simulink model "L20MSDsim"  (R2021b)
settings: Solver=FixedStepAuto  StartTime=0.0  StopTime=10  FixedStep=0.01  RelTol=1e-3
InitFcn:
  | L20ParametersMSD;
values from neighbouring files (symbols this model uses):
  A = [0 1 ; -k/m -b/m]    [L20ParametersMSD.m]    (also in L20ParametersPend.m = [0 1 ; g/l -r/(m*l^2)])
  B = [0 ; 1/m]    [L20ParametersMSD.m]    (also in L20ParametersPend.m = [0 ; 1/(m*l^2)])
  C = [1 0]    [L20ParametersMSD.m]    (also in L20ParametersPend.m)
  eta0 = -L*x0(1)    [L20ParametersMSD.m]    (also in L20ParametersPend.m)
  L = place(A(2,2),A(1,2),-10)    [L20ParametersMSD.m]    (also in L20ParametersPend.m = place(A(2,2),A(1,2),-2))
  x0 = [1; 0.5]    [L20ParametersMSD.m]    (also in L20ParametersPend.m = [theta0 ; thetadot0])
settings Model: Creator=vcichella  LastModifiedBy=vcichella_l
settings SolverCC: AlgebraicLoopSolver=TrustRegion
settings DebuggingCC: SFMachineParentedDataDiag=warning

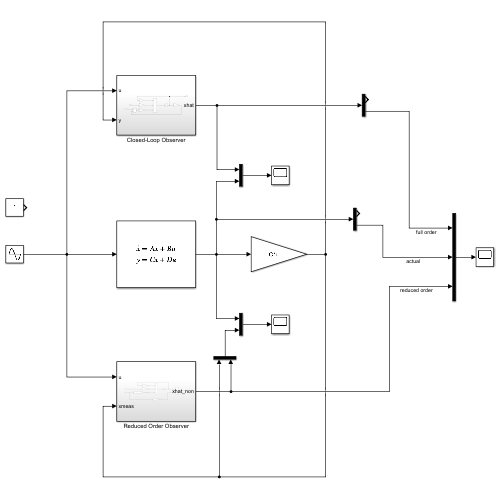
[thumbnail: Simulink's stored preview of the top-level diagram]
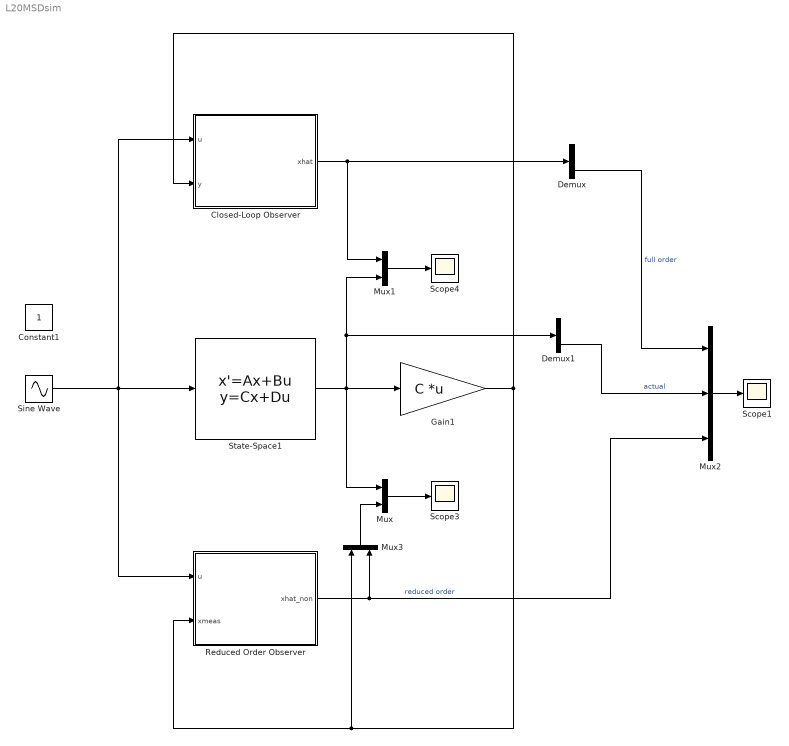
== system L20MSDsim ==
  Closed-Loop Observer : Subsystem
  Constant1 : Constant
  Demux : Demux  Outputs=2
  Demux1 : Demux  Outputs=2
  Gain1 : Gain  Gain=C  Multiplication=Matrix(K*u)
  Mux : Mux  Inputs=2
  Mux1 : Mux  Inputs=2
  Mux2 : Mux  Inputs=3
  Mux3 : Mux  Inputs=2
  Reduced Order Observer : Subsystem
  Scope1 : Scope
  Scope3 : Scope
  Scope4 : Scope
  Sine Wave : Sin  Frequency=0.1  SampleTime=0
  State-Space1 : StateSpace  A=A  B=B  C=eye(size(A))  D=zeros(2,1)  InitialCondition=x0
  wires:
  Gain1/1 -> Mux3/1, Reduced Order Observer/2(xmeas), Closed-Loop Observer/2(y)
  State-Space1/1 -> Demux1/1, Mux1/2, Mux/1, Gain1/1
  Sine Wave/1 -> Reduced Order Observer/1(u), Closed-Loop Observer/1(u), State-Space1/1
  Mux/1 -> Scope3/1
  Mux1/1 -> Scope4/1
  Closed-Loop Observer/1(xhat) -> Demux/1, Mux1/1
  Reduced Order Observer/1(xhat_non) -> Mux3/2, Mux2/3  "reduced order"
  Mux2/1 -> Scope1/1
  Demux/2 -> Mux2/1  "full order"
  Demux1/2 -> Mux2/2  "actual"
  Mux3/1 -> Mux/2

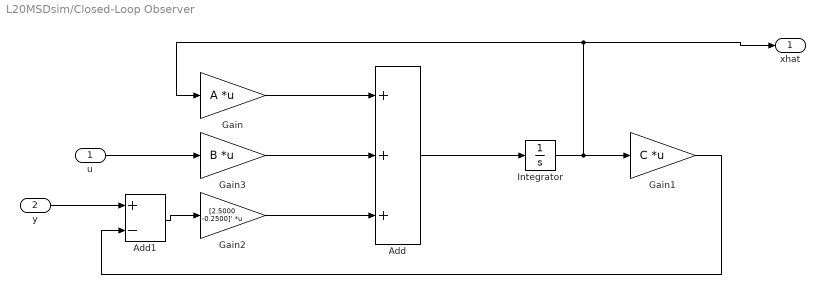
== system L20MSDsim/Closed-Loop Observer ==
  u : Inport
  y : Inport  Port=2
  Add : Sum  Inputs=+++
  Add1 : Sum  Inputs=+-
  Gain : Gain  Gain=A  Multiplication=Matrix(K*u)
  Gain1 : Gain  Gain=C  Multiplication=Matrix(K*u)
  Gain2 : Gain  Gain="[2.5000   -0.2500]'"  Multiplication=Matrix(K*u)
  Gain3 : Gain  Gain=B  Multiplication=Matrix(K*u)
  Integrator : Integrator  InitialCondition=[1;0]
  xhat : Outport
  wires:
  Add/1 -> Integrator/1
  Gain/1 -> Add/1
  Gain1/1 -> Add1/2
  Add1/1 -> Gain2/1
  y/1 -> Add1/1
  Gain2/1 -> Add/3
  u/1 -> Gain3/1
  Gain3/1 -> Add/2
  Integrator/1 -> xhat/1, Gain/1, Gain1/1

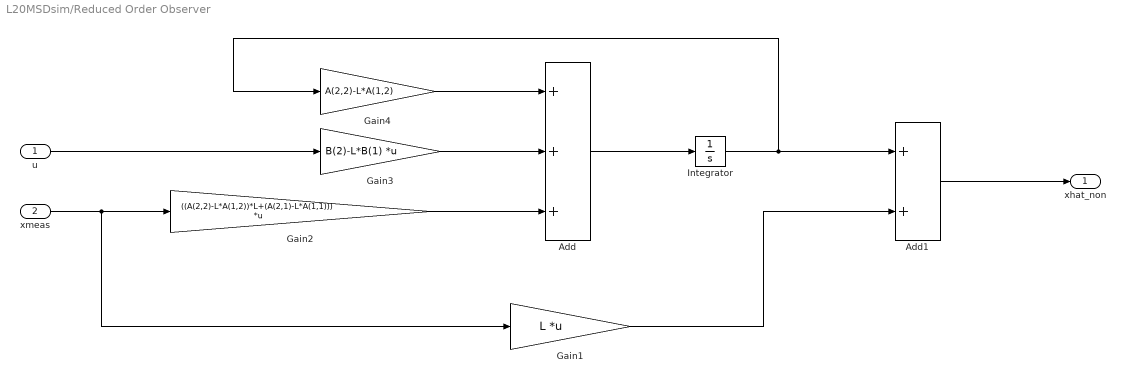
== system L20MSDsim/Reduced Order Observer ==
  u : Inport
  xmeas : Inport  Port=2
  Add : Sum  Inputs=+++
  Add1 : Sum
  Gain1 : Gain  Gain=L  Multiplication=Matrix(K*u)
  Gain2 : Gain  Gain=((A(2,2)-L*A(1,2))*L+(A(2,1)-L*A(1,1)))  Multiplication=Matrix(K*u)
  Gain3 : Gain  Gain=B(2)-L*B(1)  Multiplication=Matrix(K*u)
  Gain4 : Gain  Gain=A(2,2)-L*A(1,2)
  Integrator : Integrator  InitialCondition=eta0
  xhat_non : Outport
  wires:
  Gain3/1 -> Add/2
  u/1 -> Gain3/1
  Gain2/1 -> Add/3
  xmeas/1 -> Gain1/1, Gain2/1
  Gain4/1 -> Add/1
  Add/1 -> Integrator/1
  Integrator/1 -> Add1/1, Gain4/1
  Add1/1 -> xhat_non/1
  Gain1/1 -> Add1/2
